simulink library "linearization"  (R2016b)
settings: Solver=VariableStepAuto  StartTime=0.0  StopTime=10.0  RelTol=1e-3
undefined symbols (not defined in the file or in its folder): fsw_params, lin
libraries: aerolibutil x2, simulink_extras x1
settings Model: Creator=bijan  LastModifiedBy=bijan

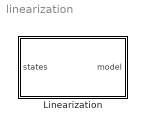
== system linearization ==
  Linearization : Subsystem

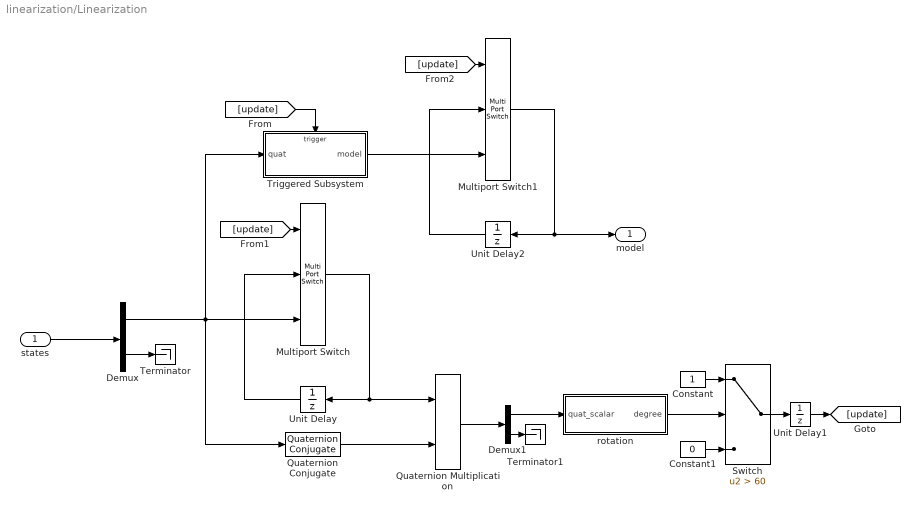
== system linearization/Linearization ==
  states : Inport
  Constant : Constant
  Constant1 : Constant  Value=0
  Demux : Demux  Outputs=[4 3]
  Demux1 : Demux  Outputs=[1 3]
  Multiport Switch : MultiPortSwitch  DataPortOrder=Zero-based contiguous  Inputs=2  DataPortIndices={0,1}
  Multiport Switch1 : MultiPortSwitch  DataPortOrder=Zero-based contiguous  Inputs=2  DataPortIndices={0,1}
  Quaternion Conjugate : aerolibutil/Quaternion Conjugate
  Quaternion Multiplication : aerolibutil/Quaternion Multiplication
  Switch : Switch  Criteria=u2 > Threshold  Threshold=60
  Terminator : Terminator
  Terminator1 : Terminator
  Triggered Subsystem : Subsystem  TreatAsAtomicUnit=on
  Unit Delay : UnitDelay  InitialCondition=[1 0 0 0]  SampleTime=-1
  Unit Delay1 : UnitDelay  SampleTime=-1
  Unit Delay2 : UnitDelay  InitialCondition=lin.bus_ic  SampleTime=-1
  rotation : Subsystem
  model : Outport
  wires:
  states/1 -> Demux/1
  Demux/2 -> Terminator/1
  Demux/1 -> Triggered Subsystem/1(quat), Quaternion Conjugate/1, Multiport Switch/3
  Multiport Switch/1 -> Unit Delay/1, Quaternion Multiplication/1
  Unit Delay/1 -> Multiport Switch/2
  Quaternion Conjugate/1 -> Quaternion Multiplication/2
  Quaternion Multiplication/1 -> Demux1/1
  Demux1/2 -> Terminator1/1
  Demux1/1 -> rotation/1(quat_scalar)
  rotation/1(degree) -> Switch/2
  Constant/1 -> Switch/1
  Constant1/1 -> Switch/3
  Switch/1 -> Unit Delay1/1
  [update] -> Triggered Subsystem/Trigger
  [update] -> Multiport Switch/1
  Unit Delay1/1 -> [update]
  Unit Delay2/1 -> Multiport Switch1/2
  Triggered Subsystem/1(model) -> Multiport Switch1/3
  Multiport Switch1/1 -> model/1, Unit Delay2/1
  [update] -> Multiport Switch1/1

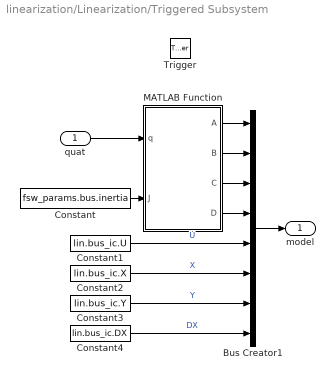
== system linearization/Linearization/Triggered Subsystem ==
  quat : Inport
  Trigger : TriggerPort  VariantControl=Variant
  Bus Creator1 : BusCreator  Inputs=8
  Constant : Constant  Value=fsw_params.bus.inertia
  Constant1 : Constant  Value=lin.bus_ic.U
  Constant2 : Constant  Value=lin.bus_ic.X
  Constant3 : Constant  Value=lin.bus_ic.Y
  Constant4 : Constant  Value=lin.bus_ic.DX
  MATLAB Function : MATLAB Function  TreatAsAtomicUnit=on
  model : Outport
  wires:
  quat/1 -> MATLAB Function/1(q)
  Constant/1 -> MATLAB Function/2(J)
  MATLAB Function/1(A) -> Bus Creator1/1
  MATLAB Function/2(B) -> Bus Creator1/2
  MATLAB Function/3(C) -> Bus Creator1/3
  MATLAB Function/4(D) -> Bus Creator1/4
  Constant1/1 -> Bus Creator1/5  "U"
  Constant2/1 -> Bus Creator1/6  "X"
  Constant3/1 -> Bus Creator1/7  "Y"
  Constant4/1 -> Bus Creator1/8  "DX"
  Bus Creator1/1 -> model/1

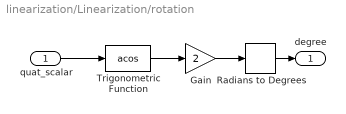
== system linearization/Linearization/rotation ==
  quat_scalar : Inport
  Gain : Gain  Gain=2
  Radians to Degrees : simulink_extras/Transformations/Radians to Degrees
  Trigonometric Function : Trigonometry  Operator=acos
  degree : Outport
  wires:
  Gain/1 -> Radians to Degrees/1
  Radians to Degrees/1 -> degree/1
  quat_scalar/1 -> Trigonometric Function/1
  Trigonometric Function/1 -> Gain/1

== matlab function linearization/Linearization/Triggered Subsystem/MATLAB Function ==
  data: q input; A output; J input; B output; C output; D output
function [A, B, C, D] = linearization(q, J)


XIq     = [ q(1) -q(2) -q(3);
            q(2)  q(1) -q(4);
            q(3)  q(4)  q(1);
            q(4) -q(2)  q(2) ];

AA = [ zeros(4) 0.5*XIq;
        zeros(3,4) zeros(3) ];

J_inv = inv(J);
B = Delta*[zeros(4,3); J_inv];
A = Delta*AA + eye(Nx);
C = eye(Nx);
D = zeros(7,3);
